simulink model "LedsSenal_prototipo"  (R2022b)
settings: Solver=VariableStepAuto  StartTime=0.0  StopTime=10.0  RelTol=1e-3
libraries: arduinolib x3, simulink x3
settings Model: Creator=dar.io  LastModifiedBy=dar.io

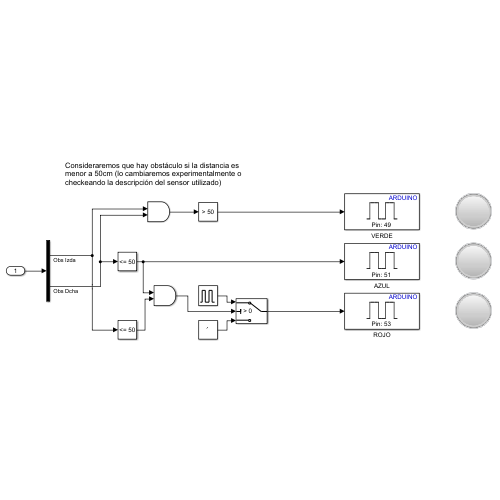
[thumbnail: Simulink's stored preview of the top-level diagram]
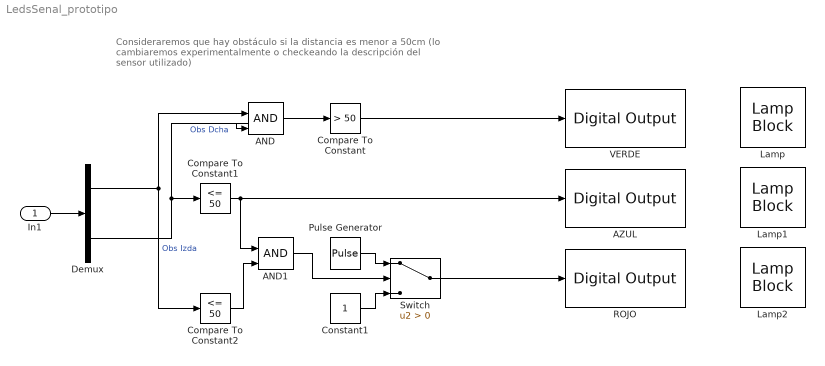
== system LedsSenal_prototipo ==
  note: Consideraremos que hay obstáculo si la distancia es menor a 50cm (lo cambiaremos experimentalmente o checkeando la descripción del sensor utilizado)
  In1 : Inport
  AND : Logic  IconShape=distinctive  AllPortsSameDT=off  OutDataTypeStr=boolean
  AND1 : Logic  IconShape=distinctive  AllPortsSameDT=off  OutDataTypeStr=boolean
  AZUL : arduinolib/Digital Output  pinNumber=51  Direction=output  blockPlatform=arduino
  Compare To Constant : simulink/Logic and Bit Operations/Compare To Constant  relop=>  const=50  OutDataTypeStr=boolean
  Compare To Constant1 : simulink/Logic and Bit Operations/Compare To Constant  relop=<=  const=50  OutDataTypeStr=boolean
  Compare To Constant2 : simulink/Logic and Bit Operations/Compare To Constant  relop=<=  const=50  OutDataTypeStr=boolean
  Constant1 : Constant
  Demux : Demux  Outputs=2
  Lamp : LampBlock  LabelPosition=Hide
  Lamp1 : LampBlock  LabelPosition=Hide
  Lamp2 : LampBlock  LabelPosition=Hide
  Pulse Generator : DiscretePulseGenerator  PulseType=Time based  Period=1  PulseWidth=50
  ROJO : arduinolib/Digital Output  pinNumber=53  Direction=output  blockPlatform=arduino
  Switch : Switch  Criteria=u2 > Threshold  SaturateOnIntegerOverflow=off  InputSameDT=off
  VERDE : arduinolib/Digital Output  pinNumber=49  Direction=output  blockPlatform=arduino
  wires:
  Compare To Constant1/1 -> AZUL/1, AND1/1
  Compare To Constant/1 -> VERDE/1
  Switch/1 -> ROJO/1
  Demux/1 -> Compare To Constant2/1, AND/1  "Obs Izda"
  Demux/2 -> Compare To Constant1/1, AND/2  "Obs Dcha"
  AND/1 -> Compare To Constant/1
  Pulse Generator/1 -> Switch/1
  Constant1/1 -> Switch/3
  AND1/1 -> Switch/2
  Compare To Constant2/1 -> AND1/2
  In1/1 -> Demux/1
